simulink model "q1"  (R2018a)
settings: Solver=FixedStepAuto  StartTime=0.0  StopTime=10.0  FixedStep=0.00001  RelTol=1e-3
settings Model: Creator=hp  LastModifiedBy=hp
settings ConfigComp: CovScope=ReferencedModels  CovIncludeTopModel=off

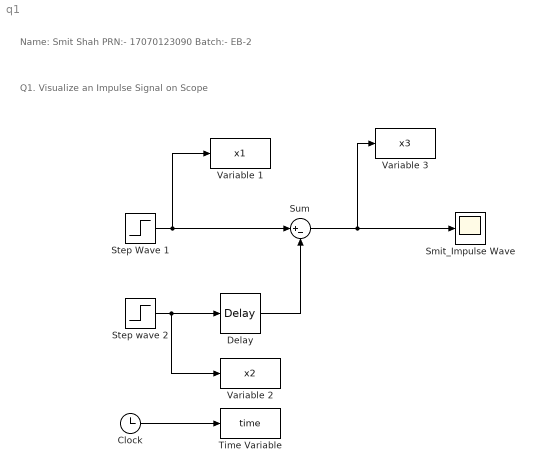
== system q1 ==
  note: Q1. Visualize an Impulse Signal on Scope
  note: Name: Smit Shah PRN:- 17070123090 Batch:- EB-2
  "Clock " : Clock
  Delay : TransportDelay  DelayTime=0.00001
  Smit_Impulse Wave : Scope
  Step Wave 1 : Step  Time=0  SampleTime=0
  Step wave 2 : Step  Time=0  After=2  SampleTime=0
  Sum : Sum  Inputs=|+-
  Time Variable : ToWorkspace  VariableName=time  SampleTime=-1
  Variable 1 : ToWorkspace  VariableName=x1  SampleTime=-1
  Variable 2 : ToWorkspace  VariableName=x2  SampleTime=-1
  Variable 3 : ToWorkspace  VariableName=x3  SampleTime=-1
  wires:
  Step Wave 1/1 -> Sum/1, Variable 1/1
  Step wave 2/1 -> Variable 2/1, Delay/1
  "Clock "/1 -> Time Variable/1
  Delay/1 -> Sum/2
  Sum/1 -> Variable 3/1, Smit_Impulse Wave/1
